simulink model "sampleModel1872"  (R2023a)
settings: Solver=VariableStepAuto  StartTime=0.0  StopTime=10.0  RelTol=1e-3
libraries: hdlsllib x5, simulink x2
settings Model: Creator=user1  LastModifiedBy=user1

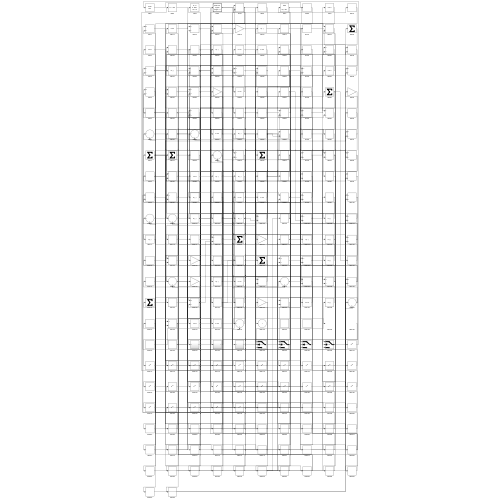
[thumbnail: Simulink's stored preview of the top-level diagram]
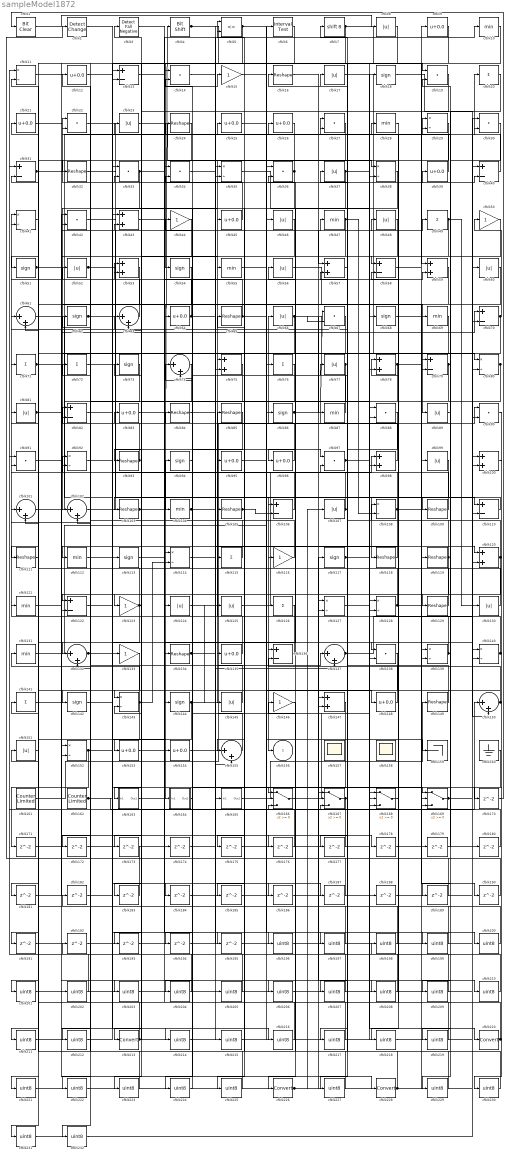
== system sampleModel1872 ==
  cfblk1 : simulink/Logic and Bit Operations/Bit Clear  iBit=0
      settings: LibrarySourceBlock=|
      | hdlsllib/Logic and Bit
      | Operations/Bit Clear
  cfblk{10,28,47,55,69,87,104,112,121,131} (10 alike) : MinMax
  cfblk{43,53,57,59,75,78,98,100,120,147} (10 alike) : Sum
  cfblk{61,63,74,101..102,132,137,150,155} (9 alike) : Sum  Inputs=|++
  cfblk{16,24,32,65,84..85,93,103,105,109,111,118..119,129,134,149} (16 alike) : Reshape
  cfblk{13,31,40,58,70,79,82,106,110,122,136} (11 alike) : Sum  Inputs=+-
  cfblk{8,17,23,37,46,48,52,56,60,66,77,81,89,99,107,124..125,130,145,151} (20 alike) : Abs  SaturateOnIntegerOverflow=off
  cfblk{11,29,35,38,41,80,92,108,114,127..128,139..140,143,152} (15 alike) : Product  Inputs=*/  RndMeth=Zero  SaturateOnIntegerOverflow=on
  cfblk{18,51,54,62,68,73,86,94,113,117,142,144} (12 alike) : Signum
  cfblk{20,49,71..72,76,115,126,141} (8 alike) : Sum  Inputs=+
  cfblk{15,44,50,116,123,133,146} (7 alike) : Gain
  cfblk{9,12,21,25..26,39,45,64,83,95..96,135,148,153..154} (15 alike) : Bias  Bias=0.0  SaturateOnIntegerOverflow=off
  cfblk{14,19,22,27,30,33..34,36,42,67,88,90..91,97,138} (15 alike) : DotProduct  OutDataTypeStr=Inherit: Inherit via internal rule
  cfblk157 : Scope
      settings: Floating=on
  cfblk158 : Scope
      settings: Floating=on
  cfblk159 : Terminator
  cfblk160 : Ground
  cfblk161 : hdlsllib/Sources/Counter Limited  uplimit=7  tsamp=-1
  cfblk162 : hdlsllib/Sources/Counter Limited  uplimit=7  tsamp=-1
  cfblk163 : Subsystem
      settings: LibrarySourceBlock=|
      | hdlsllib/Ports &
      | Subsystems/Subsystem
  cfblk164 : Subsystem
      settings: LibrarySourceBlock=|
      | hdlsllib/Ports &
      | Subsystems/Subsystem
  cfblk165 : Subsystem
      settings: LibrarySourceBlock=|
      | hdlsllib/Ports &
      | Subsystems/Subsystem
  cfblk{166..169} (4 alike) : Switch  SaturateOnIntegerOverflow=off  InputSameDT=off
  cfblk{170..195} (26 alike) : Delay  SampleTime=1
  cfblk{196..212,214..219,221..225,227,229..232} (33 alike) : DataTypeConversion  OutDataTypeStr=uint8  SaturateOnIntegerOverflow=off  RndMeth=Floor
  cfblk2 : simulink/Logic and Bit Operations/Detect Change  vinit=0  OutDataTypeStr=boolean
      settings: LibrarySourceBlock=|
      | hdlsllib/Logic and Bit
      | Operations/Detect
      | Change
  cfblk{213,220,226,228} (4 alike) : DataTypeConversion  SaturateOnIntegerOverflow=off  RndMeth=Floor
  cfblk3 : hdlsllib/Logic and Bit Operations/Detect Fall Negative  vinit=0  OutDataTypeStr=boolean
  cfblk4 : hdlsllib/Logic and Bit Operations/Bit Shift  mode=Shift Left Logical  N=0
  cfblk5 : RelationalOperator  Operator=<=  OutDataTypeStr=boolean  InputSameDT=off
  cfblk6 : hdlsllib/Logic and Bit Operations/Interval Test  IntervalClosedRight=on  uplimit=0.5  IntervalClosedLeft=on  lowlimit=-0.5  OutDataTypeStr=boolean
  cfblk7 : ArithShift  BitShiftNumber=8
  cfblk156 : Outport  VectorParamsAs1DForOutWhenUnconnected=off
  wires:
  cfblk161/1 -> cfblk137/1
  cfblk124/1 -> cfblk90/1
  cfblk102/1 -> cfblk47/1
  cfblk167/1 -> cfblk41/1, cfblk166/3
  cfblk62/1 -> cfblk97/1, cfblk64/1
  cfblk144/1 -> cfblk98/1, cfblk125/1, cfblk231/1
  cfblk110/1 -> cfblk103/1
  cfblk44/1 -> cfblk153/1
  cfblk145/1 -> cfblk101/1
  cfblk27/1 -> cfblk145/1
  cfblk98/1 -> cfblk66/1
  cfblk54/1 -> cfblk164/1(In1)
  cfblk19/1 -> cfblk123/1
  cfblk103/1 -> cfblk4/1, cfblk139/2
  cfblk106/1 -> cfblk71/1
  cfblk45/1 -> cfblk22/1
  cfblk119/1 -> cfblk27/1, cfblk185/1
  cfblk60/1 -> cfblk89/1
  cfblk9/1 -> cfblk54/1
  cfblk17/1 -> cfblk79/1
  cfblk148/1 -> cfblk61/1
  cfblk22/1 -> cfblk156/1
  cfblk140/1 -> cfblk85/1, cfblk57/2
  cfblk23/1 -> cfblk38/1
  cfblk57/1 -> cfblk7/1
  cfblk128/1 -> cfblk56/1, cfblk190/1
  cfblk154/1 -> cfblk18/1
  cfblk99/1 -> cfblk124/1
  cfblk72/1 -> cfblk118/1
  cfblk42/1 -> cfblk75/1
  cfblk76/1 -> cfblk163/1(In1)
  cfblk107/1 -> cfblk21/1, cfblk177/1
  cfblk101/1 -> cfblk29/1
  cfblk164/1(Out1) -> cfblk94/1
  cfblk149/1 -> cfblk16/1
  cfblk50/1 -> cfblk58/1
  cfblk33/1 -> cfblk102/1, cfblk5/2, cfblk187/1
  cfblk139/1 -> cfblk63/1, cfblk209/1
  cfblk109/1 -> cfblk37/1
  cfblk47/1 -> cfblk96/1, cfblk108/2
  cfblk163/1(Out1) -> cfblk26/1
  cfblk162/1 -> cfblk150/1, cfblk25/1
  cfblk168/1 -> cfblk78/1
  cfblk4/1 -> cfblk35/2, cfblk138/2
  cfblk104/1 -> cfblk165/1(In1), cfblk137/2
  cfblk37/1 -> cfblk128/2, cfblk134/1, cfblk106/1, cfblk232/1
  cfblk41/1 -> cfblk61/2
  cfblk116/1 -> cfblk24/1
  cfblk52/1 -> cfblk76/1, cfblk122/1
  cfblk48/1 -> cfblk115/1
  cfblk64/1 -> cfblk41/2, cfblk138/1
  cfblk166/1 -> cfblk88/1
  cfblk94/1 -> cfblk144/1
  cfblk36/1 -> cfblk155/1, cfblk32/1
  cfblk134/1 -> cfblk44/1, cfblk169/2
  cfblk132/1 -> cfblk167/2, cfblk200/1
  cfblk165/1(Out1) -> cfblk149/1
  cfblk93/1 -> cfblk83/1, cfblk72/1
  cfblk25/1 -> cfblk88/2
  cfblk108/1 -> cfblk5/1, cfblk30/2, cfblk183/1
  cfblk30/1 -> cfblk169/1
  cfblk127/1 -> cfblk220/1
  cfblk38/1 -> cfblk136/1
  cfblk77/1 -> cfblk114/1, cfblk166/2
  cfblk58/1 -> cfblk9/1
  cfblk86/1 -> cfblk67/1, cfblk49/1
  cfblk141/1 -> cfblk228/1
  cfblk130/1 -> cfblk73/1
  cfblk131/1 -> cfblk86/1
  cfblk71/1 -> cfblk167/1, cfblk176/1, cfblk214/1
  cfblk155/1 -> cfblk84/1
  cfblk63/1 -> cfblk52/1
  cfblk55/1 -> cfblk48/1
  cfblk160/1 -> cfblk166/1
  cfblk146/1 -> cfblk226/1
  cfblk120/1 -> cfblk87/1, cfblk152/2, cfblk108/1
  cfblk87/1 -> cfblk23/1
  cfblk40/1 -> cfblk20/1
  cfblk123/1 -> cfblk31/2, cfblk53/1, cfblk221/1
  cfblk18/1 -> cfblk150/2
  cfblk80/1 -> cfblk169/3, cfblk189/1
  cfblk150/1 -> cfblk136/2, cfblk142/1
  cfblk70/1 -> cfblk50/1, cfblk225/1
  cfblk143/1 -> cfblk131/1, cfblk114/2, cfblk193/1, cfblk222/1
  cfblk89/1 -> cfblk129/1
  cfblk46/1 -> cfblk93/1
  cfblk51/1 -> cfblk69/1, cfblk80/2
  cfblk122/1 -> cfblk154/1
  cfblk78/1 -> cfblk104/1, cfblk80/1
  cfblk125/1 -> cfblk38/2
  cfblk12/1 -> cfblk19/1
  cfblk84/1 -> cfblk120/1
  cfblk10/1 -> cfblk111/1
  cfblk61/1 -> cfblk113/1
  cfblk95/1 -> cfblk110/1
  cfblk56/1 -> cfblk139/1
  cfblk7/1 -> cfblk59/1, cfblk132/1
  cfblk35/1 -> cfblk168/1
  cfblk136/1 -> cfblk135/1
  cfblk152/1 -> cfblk95/1, cfblk171/1
  cfblk1/1 -> cfblk8/1
  cfblk79/1 -> cfblk116/1, cfblk229/1
  cfblk16/1 -> cfblk57/1
  cfblk68/1 -> cfblk119/1
  cfblk32/1 -> cfblk45/1
  cfblk15/1 -> cfblk148/1
  cfblk83/1 -> cfblk59/2
  cfblk66/1 -> cfblk101/2, cfblk79/2, cfblk67/2, cfblk210/1
  cfblk13/1 -> cfblk109/1
  cfblk105/1 -> cfblk106/2, cfblk175/1
  cfblk169/1 -> cfblk40/1, cfblk29/2
  cfblk137/1 -> cfblk17/1, cfblk70/2
  cfblk75/1 -> cfblk143/1
  cfblk96/1 -> cfblk82/1
  cfblk97/1 -> cfblk77/1, cfblk40/2
  cfblk2/1 -> cfblk140/2
  cfblk24/1 -> cfblk42/2
  cfblk65/1 -> cfblk126/1, cfblk159/1, cfblk53/2
  cfblk39/1 -> cfblk22/2
  cfblk114/1 -> cfblk10/1
  cfblk135/1 -> cfblk82/2
  cfblk117/1 -> cfblk68/1, cfblk97/2
  cfblk153/1 -> cfblk39/1
  cfblk6/1 -> cfblk213/1
  cfblk115/1 -> cfblk92/1
  cfblk5/1 -> cfblk92/2, cfblk122/2, cfblk197/1
  cfblk69/1 -> cfblk105/1
  cfblk26/1 -> cfblk51/1
  cfblk49/1 -> cfblk63/2, cfblk130/1
  cfblk129/1 -> cfblk62/1
  cfblk118/1 -> cfblk112/1
  cfblk81/1 -> cfblk70/1, cfblk43/2
  cfblk43/1 -> cfblk15/1
  cfblk31/1 -> cfblk13/2, cfblk55/1
  cfblk67/1 -> cfblk147/2
  cfblk90/1 -> cfblk170/1
  cfblk170/1 -> cfblk1/1
  cfblk171/1 -> cfblk155/2
  cfblk59/1 -> cfblk172/1
  cfblk172/1 -> cfblk35/1
  cfblk29/1 -> cfblk173/1
  cfblk173/1 -> cfblk2/1
  cfblk113/1 -> cfblk174/1
  cfblk175/1 -> cfblk168/2
  cfblk176/1 -> cfblk13/1
  cfblk177/1 -> cfblk31/1
  cfblk21/1 -> cfblk178/1
  cfblk178/1 -> cfblk140/1
  cfblk179/1 -> cfblk19/2
  cfblk180/1 -> cfblk167/3
  cfblk111/1 -> cfblk181/1
  cfblk181/1 -> cfblk42/1
  cfblk183/1 -> cfblk152/1
  cfblk92/1 -> cfblk184/1
  cfblk184/1 -> cfblk128/1
  cfblk185/1 -> cfblk147/1
  cfblk142/1 -> cfblk186/1
  cfblk186/1 -> cfblk78/2
  cfblk187/1 -> cfblk143/2
  cfblk188/1 -> cfblk110/2
  cfblk189/1 -> cfblk58/2
  cfblk190/1 -> cfblk132/2
  cfblk53/1 -> cfblk191/1
  cfblk191/1 -> cfblk120/2
  cfblk192/1 -> cfblk98/2
  cfblk193/1 -> cfblk75/2
  cfblk126/1 -> cfblk194/1
  cfblk194/1 -> cfblk168/3
  cfblk112/1 -> cfblk195/1
  cfblk195/1 -> cfblk46/1
  cfblk34/1 -> cfblk196/1
  cfblk196/1 -> cfblk117/1
  cfblk197/1 -> cfblk34/1
  cfblk198/1 -> cfblk34/2
  cfblk3/1 -> cfblk199/1
  cfblk199/1 -> cfblk81/1
  cfblk200/1 -> cfblk3/1
  cfblk151/1 -> cfblk201/1
  cfblk201/1 -> cfblk60/1
  cfblk121/1 -> cfblk202/1
  cfblk202/1 -> cfblk151/1
  cfblk11/1 -> cfblk203/1
  cfblk203/1 -> cfblk36/1
  cfblk85/1 -> cfblk204/1
  cfblk204/1 -> cfblk11/1
  cfblk174/1 -> cfblk205/1
  cfblk205/1 -> cfblk11/2
  cfblk182/1 -> cfblk206/1
  cfblk206/1 -> cfblk36/2
  cfblk138/1 -> cfblk207/1
  cfblk207/1 -> cfblk182/1
  cfblk91/1 -> cfblk208/1
  cfblk208/1 -> cfblk43/1
  cfblk209/1 -> cfblk91/1
  cfblk210/1 -> cfblk91/2
  cfblk133/1 -> cfblk211/1
  cfblk211/1 -> cfblk33/1
  cfblk73/1 -> cfblk212/1
  cfblk212/1 -> cfblk133/1
  cfblk213/1 -> cfblk188/1, cfblk33/2, cfblk121/1
  cfblk214/1 -> cfblk6/1
  cfblk14/1 -> cfblk215/1
  cfblk215/1 -> cfblk99/1
  cfblk82/1 -> cfblk216/1
  cfblk216/1 -> cfblk14/1
  cfblk8/1 -> cfblk217/1
  cfblk217/1 -> cfblk14/2
  cfblk28/1 -> cfblk218/1
  cfblk218/1 -> cfblk90/2
  cfblk20/1 -> cfblk219/1
  cfblk219/1 -> cfblk28/1
  cfblk220/1 -> cfblk198/1, cfblk192/1, cfblk30/1
  cfblk221/1 -> cfblk127/1
  cfblk222/1 -> cfblk127/2
  cfblk74/1 -> cfblk223/1
  cfblk223/1 -> cfblk12/1
  cfblk147/1 -> cfblk224/1
  cfblk224/1 -> cfblk74/1
  cfblk225/1 -> cfblk74/2
  cfblk226/1 -> cfblk180/1, cfblk179/1, cfblk107/1
  cfblk88/1 -> cfblk227/1
  cfblk227/1 -> cfblk146/1
  cfblk228/1 -> cfblk27/2, cfblk65/1
  cfblk229/1 -> cfblk141/1
  cfblk100/1 -> cfblk230/1
  cfblk230/1 -> cfblk102/2
  cfblk231/1 -> cfblk100/1
  cfblk232/1 -> cfblk100/2

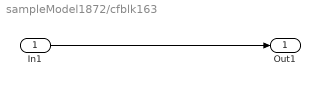
== system sampleModel1872/cfblk163 ==
  In1 : Inport
  Out1 : Outport
  wires:
  In1/1 -> Out1/1

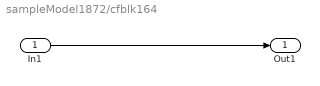
== system sampleModel1872/cfblk164 ==
  In1 : Inport
  Out1 : Outport
  wires:
  In1/1 -> Out1/1

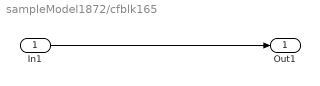
== system sampleModel1872/cfblk165 ==
  In1 : Inport
  Out1 : Outport
  wires:
  In1/1 -> Out1/1
